simulink model "Boat_model_paper"  (Simulink 6.6)
settings: Solver=ode3  StartTime=0.0  StopTime=500  FixedStep=.01  RelTol=1e-3
values from neighbouring files (symbols this model uses):
  C_d_sea_surge = -340    [boat_constants.m]
  C_F = 1.15    [boat_constants.m]
  C_T = 6.4/(pi*rho_w*rudder_span*d_prop)    (= 0.00946194530212)    [boat_constants.m]
  d_prop = .4572    (= 0.4572)    [boat_constants.m]
  delta_stall = .279    (= 0.279)    [boat_constants.m]
  e_0 = 0    [boat_constants.m]
  I_xx = mass/12*(3^2+4^2)    (= 1145.83333333)    [boat_constants.m]
  I_zz = mass/12*(13^2+3^2)    (= 8158.33333333)    [boat_constants.m]
  K_t = 0.5    [boat_constants.m]
  mass = 550    [boat_constants.m]
  n_0 = 0    [boat_constants.m]
  proportional_band = .5    (= 0.5)    [boat_constants.m]
  psi_0 = 0    [boat_constants.m]
  rho_w = 1.03e3    (= 1030)    [boat_constants.m]
  rudder_angle_dot_max = 10    [boat_constants.m]
  rudder_angle_max = 1    [boat_constants.m]
  rudder_area = .0945    (= 0.0945)    [boat_constants.m]
  Wf = 1 - Wt    (= 0.9)    [boat_constants.m]
  x_cg = .0508    (= 0.0508)    [boat_constants.m]
  x_cp = 3.4224    [boat_constants.m]
  z_cg = .0508    (= 0.0508)    [boat_constants.m]
  z_cp = .2032    (= 0.2032)    [boat_constants.m]
undefined symbols (not defined in the file or in its folder): render_boat
libraries: simulink x4, vrlib x1
settings Model: Creator=Administrator  LastModifiedBy=Administrator  SimulationMode=accelerator
settings DebuggingCC: AlgebraicLoopMsg=error

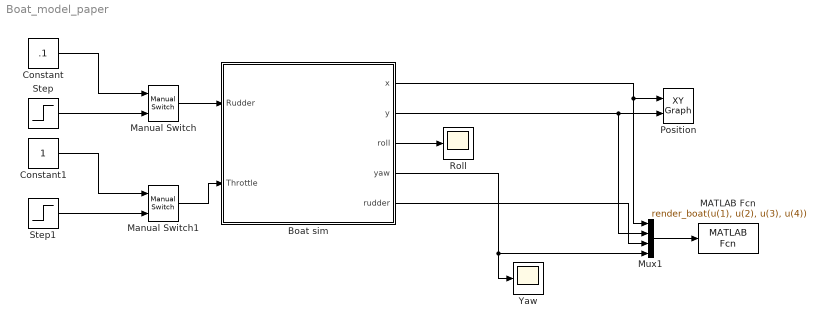
== system Boat_model_paper ==
  Boat sim : Subsystem
  Constant : Constant  Value=.1
  Constant1 : Constant
  MATLAB Fcn : MATLABFcn  MATLABFcn=render_boat(u(1), u(2), u(3), u(4))  OutputDimensions=0
  Manual Switch : simulink/Signal Routing/Manual Switch  SystemSampleTime=-1  sw=1  action=0  varsize=off
  Manual Switch1 : simulink/Signal Routing/Manual Switch  SystemSampleTime=-1  sw=1  action=0  varsize=off
  Mux1 : Mux
  Position : simulink/Sinks/XY Graph  SystemSampleTime=-1  xmin=-1000  xmax=1000  ymin=-1000  ymax=1000  st=-1
  Roll : Scope
  Step : Step  Time=5  SampleTime=0
  Step1 : Step  Time=5  SampleTime=0
  Yaw : Scope
      settings: SaveName=ScopeData4
  wires:
  Mux1/1 -> MATLAB Fcn/1
  Boat sim/1(x) -> Mux1/1, Position/1
  Boat sim/2(y) -> Position/2, Mux1/2
  Boat sim/4(yaw) -> Mux1/4, Yaw/1
  Boat sim/3(roll) -> Roll/1
  Boat sim/5(rudder) -> Mux1/3
  Step/1 -> Manual Switch/2
  Manual Switch/1 -> Boat sim/1(Rudder)
  Constant/1 -> Manual Switch/1
  Step1/1 -> Manual Switch1/2
  Manual Switch1/1 -> Boat sim/2(Throttle)
  Constant1/1 -> Manual Switch1/1

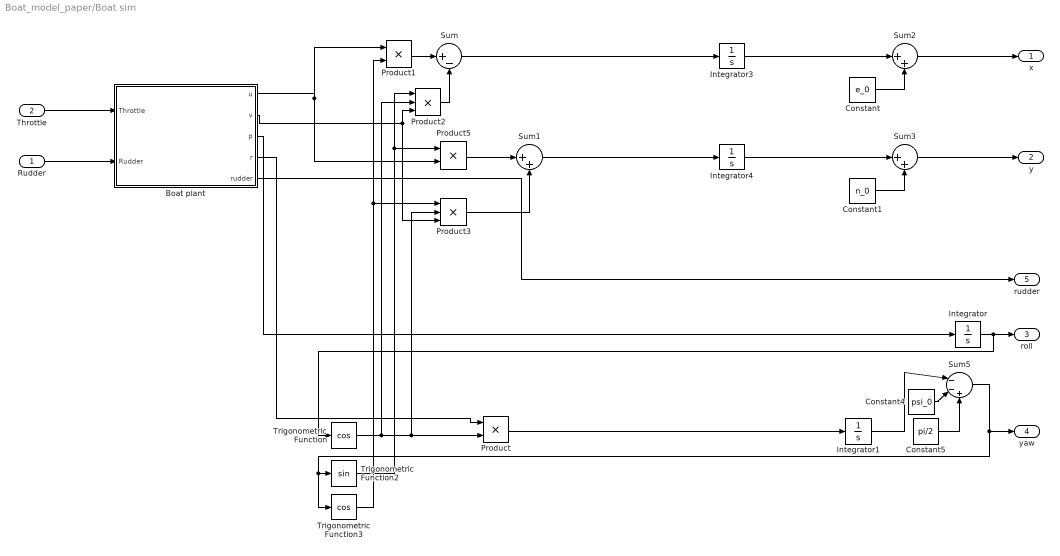
== system Boat_model_paper/Boat sim ==
  Rudder : Inport
  Throttle : Inport  Port=2
  Boat plant : Subsystem
  Constant : Constant  Value=e_0
  Constant1 : Constant  Value=n_0
  Constant4 : Constant  Value=psi_0
  Constant5 : Constant  Value=pi/2
  Integrator{,1,3..4} (4 alike) : Integrator
  Product : Product  RndMeth=Zero
  Product1 : Product  RndMeth=Zero
  Product2 : Product  Inputs=3  RndMeth=Zero
  Product3 : Product  Inputs=3  RndMeth=Zero
  Product5 : Product  RndMeth=Zero
  Sum : Sum  Inputs=|+-
  Sum1 : Sum  Inputs=|++
  Sum2 : Sum  Inputs=|++
  Sum3 : Sum  Inputs=|++
  Sum5 : Sum  Inputs=|--+
  Trigonometric Function : Trigonometry  Operator=cos
  Trigonometric Function2 : Trigonometry
  Trigonometric Function3 : Trigonometry  Operator=cos
  x : Outport
  y : Outport  Port=2
  roll : Outport  Port=3
  yaw : Outport  Port=4
  rudder : Outport  Port=5
  wires:
  Throttle/1 -> Boat plant/1(Throttle)
  Rudder/1 -> Boat plant/2(Rudder)
  Boat plant/3(p) -> Integrator/1
  Trigonometric Function/1 -> Product/2, Product3/2, Product2/2
  Boat plant/4(r) -> Product/1
  Product/1 -> Integrator1/1
  Product2/1 -> Sum/2
  Product1/1 -> Sum/1
  Boat plant/1(u) -> Product1/1, Product5/2
  Trigonometric Function3/1 -> Product1/2, Product3/1
  Trigonometric Function2/1 -> Product2/1, Product5/1
  Boat plant/2(v) -> Product2/3, Product3/3
  Product5/1 -> Sum1/1
  Product3/1 -> Sum1/2
  Sum/1 -> Integrator3/1
  Integrator/1 -> roll/1, Trigonometric Function/1
  Constant4/1 -> Sum5/2
  Constant5/1 -> Sum5/3
  Integrator1/1 -> Sum5/1
  Sum5/1 -> yaw/1, Trigonometric Function2/1, Trigonometric Function3/1
  Boat plant/5(rudder) -> rudder/1
  Constant/1 -> Sum2/2
  Integrator3/1 -> Sum2/1
  Sum2/1 -> x/1
  Integrator4/1 -> Sum3/1
  Constant1/1 -> Sum3/2
  Sum3/1 -> y/1
  Sum1/1 -> Integrator4/1

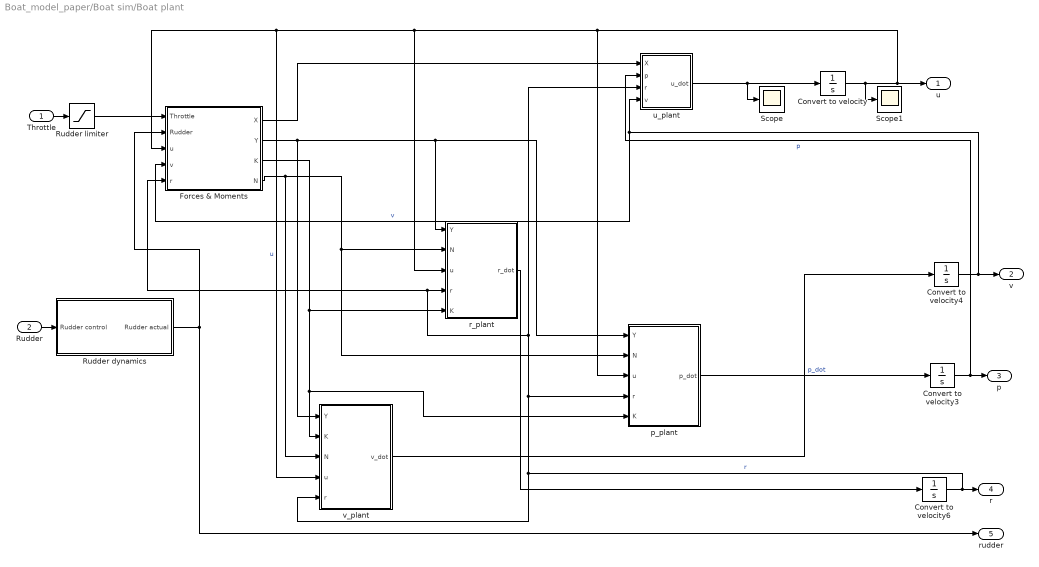
== system Boat_model_paper/Boat sim/Boat plant ==
  Throttle : Inport
  Rudder : Inport  Port=2
  Convert to velocity{,3..4,6} (4 alike) : Integrator
  Forces & Moments : Subsystem
  Rudder dynamics : Subsystem
  Rudder limiter : Saturate  UpperLimit=1  LowerLimit=0
  Scope : Scope
      settings: SaveName=ScopeData2
  Scope1 : Scope
      settings: SaveName=ScopeData3
  p_plant : Subsystem
  r_plant : Subsystem
  u_plant : Subsystem
  v_plant : Subsystem
  u : Outport
  v : Outport  Port=2
  p : Outport  Port=3
  r : Outport  Port=4
  rudder : Outport  Port=5
  wires:
  Convert to velocity/1 -> u/1, r_plant/3(u), Forces & Moments/3(u), v_plant/4(u), p_plant/3(u), Scope1/1  "u"
  Forces & Moments/1(X) -> u_plant/1(X)
  Rudder/1 -> Rudder dynamics/1(Rudder control)
  Throttle/1 -> Rudder limiter/1
  Convert to velocity4/1 -> v/1, u_plant/4(v), Forces & Moments/4(v)  "v"
  p_plant/1(p_dot) -> Convert to velocity3/1  "p_dot"
  Convert to velocity3/1 -> p/1, u_plant/2(p)  "p"
  Convert to velocity6/1 -> r/1, v_plant/5(r), u_plant/3(r), r_plant/4(r), Forces & Moments/5(r), p_plant/4(r)  "r"
  u_plant/1(u_dot) -> Convert to velocity/1, Scope/1
  Forces & Moments/4(N) -> v_plant/3(N), r_plant/2(N), p_plant/2(N)
  Forces & Moments/3(K) -> v_plant/2(K), p_plant/5(K), r_plant/5(K)
  Forces & Moments/2(Y) -> v_plant/1(Y), r_plant/1(Y), p_plant/1(Y)
  v_plant/1(v_dot) -> Convert to velocity4/1
  r_plant/1(r_dot) -> Convert to velocity6/1
  Rudder limiter/1 -> Forces & Moments/1(Throttle)
  Rudder dynamics/1(Rudder actual) -> Forces & Moments/2(Rudder), rudder/1

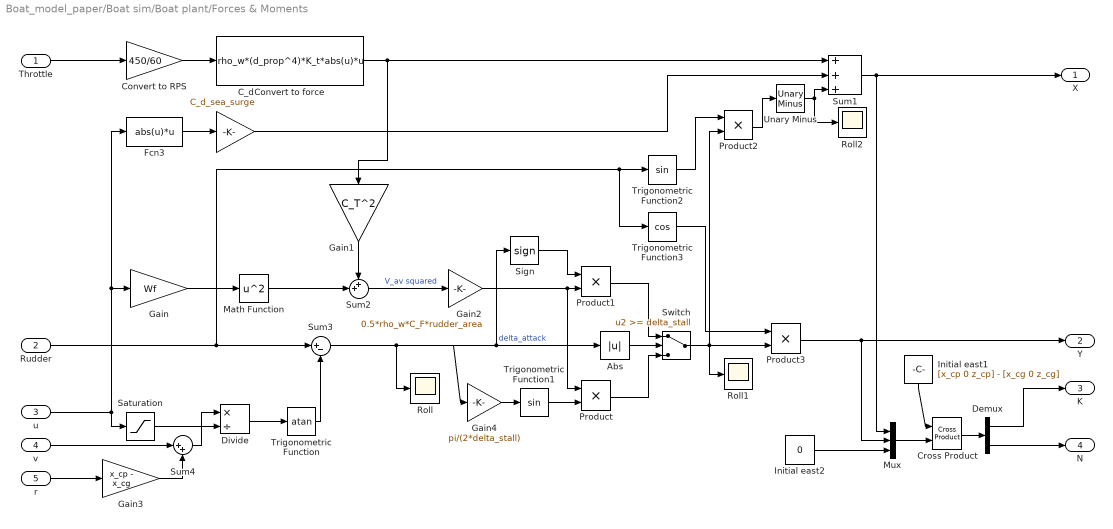
== system Boat_model_paper/Boat sim/Boat plant/Forces & Moments ==
  Throttle : Inport
  Rudder : Inport  Port=2
  u : Inport  Port=3
  v : Inport  Port=4
  r : Inport  Port=5
  Abs : Abs
  C_d : Gain  Gain=C_d_sea_surge
  Convert to RPS : Gain  Gain=450/60
  Convert to force : Fcn  Expr=rho_w*(d_prop^4)*K_t*abs(u)*u
  Cross Product : vrlib/Utilities/Cross Product  SystemSampleTime=-1
  Demux : Demux  Outputs=3
  Divide : Product  Inputs=*/  OutScaling=2^-10
  Fcn3 : Fcn  Expr=abs(u)*u
  Gain : Gain  Gain=Wf
  Gain1 : Gain  Orientation=down  Gain=C_T^2
  Gain2 : Gain  Gain=0.5*rho_w*C_F*rudder_area
  Gain3 : Gain  Gain=x_cp - x_cg
  Gain4 : Gain  Gain=pi/(2*delta_stall)
  Initial east1 : Constant  Orientation=down  Value=[x_cp 0 z_cp] - [x_cg 0 z_cg]
  Initial east2 : Constant  Value=0
  Math Function : Math  Operator=square  SaturateOnIntegerOverflow=on
  Mux : Mux  Inputs=3
  Product{,1..3} (4 alike) : Product  RndMeth=Zero
  Roll : Scope
  Roll1 : Scope
      settings: SaveName=ScopeData5
  Roll2 : Scope
      settings: SaveName=ScopeData6
  Saturation : Saturate  UpperLimit=inf  LowerLimit=0.00001
  Sign : Signum
  Sum1 : Sum  Inputs=+++
  Sum2 : Sum  Inputs=++|
  Sum3 : Sum  Inputs=|+-
  Sum4 : Sum  Inputs=|++
  Switch : Switch  Threshold=delta_stall
  Trigonometric Function : Trigonometry  Operator=atan
  Trigonometric Function1 : Trigonometry
  Trigonometric Function2 : Trigonometry
  Trigonometric Function3 : Trigonometry  Operator=cos
  Unary Minus : simulink/Math Operations/Unary Minus  DoSatur=off
  X : Outport
  Y : Outport  Port=2
  K : Outport  Port=3
  N : Outport  Port=4
  wires:
  Convert to RPS/1 -> Convert to force/1
  Fcn3/1 -> C_d/1
  C_d/1 -> Sum1/2
  Convert to force/1 -> Sum1/1, Gain1/1
  u/1 -> Fcn3/1, Gain/1, Saturation/1
  Throttle/1 -> Convert to RPS/1
  Sum1/1 -> X/1, Mux/1
  Gain/1 -> Math Function/1
  Gain1/1 -> Sum2/1
  Math Function/1 -> Sum2/2
  Sum2/1 -> Gain2/1  "V_av squared"
  Rudder/1 -> Sum3/1, Trigonometric Function2/1, Trigonometric Function3/1
  r/1 -> Gain3/1
  Gain3/1 -> Sum4/2
  v/1 -> Sum4/1
  Divide/1 -> Trigonometric Function/1
  Sum4/1 -> Divide/1
  Trigonometric Function/1 -> Sum3/2
  Sum3/1 -> Abs/1, Sign/1, Gain4/1, Roll/1  "delta_attack"
  Abs/1 -> Switch/2
  Product/1 -> Switch/3
  Trigonometric Function1/1 -> Product/2
  Gain2/1 -> Product/1, Product1/2
  Product1/1 -> Switch/1
  Sign/1 -> Product1/1
  Gain4/1 -> Trigonometric Function1/1
  Unary Minus/1 -> Sum1/3, Roll2/1
  Product2/1 -> Unary Minus/1
  Trigonometric Function2/1 -> Product2/1
  Trigonometric Function3/1 -> Product3/1
  Product3/1 -> Y/1, Mux/2
  Cross Product/1 -> Demux/1
  Demux/1 -> K/1
  Demux/3 -> N/1
  Switch/1 -> Product2/2, Product3/2, Roll1/1
  Saturation/1 -> Divide/2
  Initial east2/1 -> Mux/3
  Mux/1 -> Cross Product/2
  Initial east1/1 -> Cross Product/1

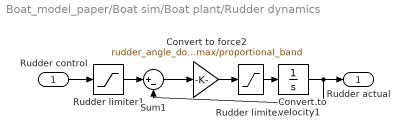
== system Boat_model_paper/Boat sim/Boat plant/Rudder dynamics ==
  Rudder control : Inport
  Convert to force2 : Gain  Gain=rudder_angle_dot_max/proportional_band
  Convert to velocity1 : Integrator  LimitOutput=on  UpperSaturationLimit=rudder_angle_max  LowerSaturationLimit=-rudder_angle_max
  Rudder limiter1 : Saturate  UpperLimit=rudder_angle_max  LowerLimit=-rudder_angle_max
  Rudder limiter2 : Saturate  UpperLimit=rudder_angle_dot_max  LowerLimit=-rudder_angle_dot_max
  Sum1 : Sum  Inputs=|+-
  Rudder actual : Outport
  wires:
  Convert to velocity1/1 -> Rudder actual/1, Sum1/2
  Sum1/1 -> Convert to force2/1
  Rudder limiter1/1 -> Sum1/1
  Rudder limiter2/1 -> Convert to velocity1/1
  Convert to force2/1 -> Rudder limiter2/1
  Rudder control/1 -> Rudder limiter1/1

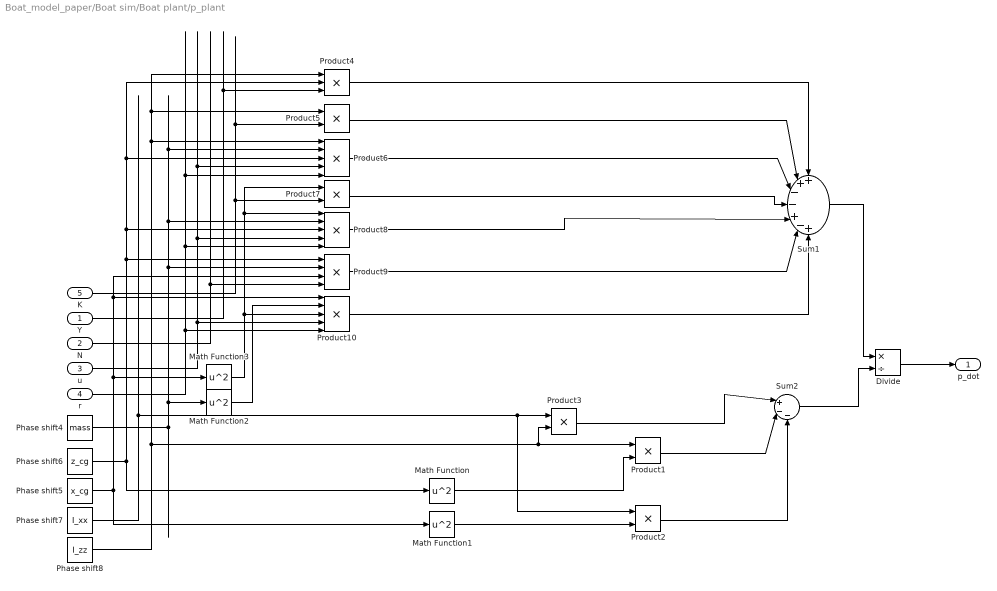
== system Boat_model_paper/Boat sim/Boat plant/p_plant ==
  Y : Inport
  N : Inport  Port=2
  u : Inport  Port=3
  r : Inport  Port=4
  K : Inport  Port=5
  Divide : Product  Inputs=*/  OutScaling=2^-10
  Math Function{,1..3} (4 alike) : Math  Operator=square  SaturateOnIntegerOverflow=on
  Phase shift4 : Constant  Value=mass
  Phase shift5 : Constant  Value=x_cg
  Phase shift6 : Constant  Value=z_cg
  Phase shift7 : Constant  Value=I_xx
  Phase shift8 : Constant  Value=I_zz
  Product{1..3,5,7} (5 alike) : Product  RndMeth=Zero
  Product10 : Product  Inputs=5  RndMeth=Zero
  Product4 : Product  Inputs=3  RndMeth=Zero
  Product6 : Product  Inputs=5  RndMeth=Zero
  Product8 : Product  Inputs=5  RndMeth=Zero
  Product9 : Product  Inputs=4  RndMeth=Zero
  Sum1 : Sum  Inputs=++--+-+
  Sum2 : Sum  Inputs=|+--
  p_dot : Outport
  wires:
  Sum1/1 -> Divide/1
  Divide/1 -> p_dot/1
  r/1 -> Product6/5, Product8/5, Product10/5
  u/1 -> Product6/4, Product8/4, Product10/4
  N/1 -> Product9/4
  Y/1 -> Product4/3
  Sum2/1 -> Divide/2
  Phase shift7/1 -> Product3/1, Product2/1
  Phase shift8/1 -> Product3/2, Product1/1, Product4/1, Product5/1, Product6/1
  Product3/1 -> Sum2/1
  Phase shift6/1 -> Math Function/1, Product4/2, Product6/3, Product8/3, Product9/1
  Math Function/1 -> Product1/2
  Product1/1 -> Sum2/2
  Math Function1/1 -> Product2/2
  Product2/1 -> Sum2/3
  Phase shift4/1 -> Product6/2, Product8/2, Product9/2, Math Function2/1
  K/1 -> Product5/2, Product7/2
  Phase shift5/1 -> Math Function1/1, Math Function3/1, Product9/3, Product10/1
  Product4/1 -> Sum1/1
  Product5/1 -> Sum1/2
  Product6/1 -> Sum1/3
  Product7/1 -> Sum1/4
  Math Function3/1 -> Product7/1, Product8/1, Product10/3
  Product8/1 -> Sum1/5
  Product9/1 -> Sum1/6
  Product10/1 -> Sum1/7
  Math Function2/1 -> Product10/2

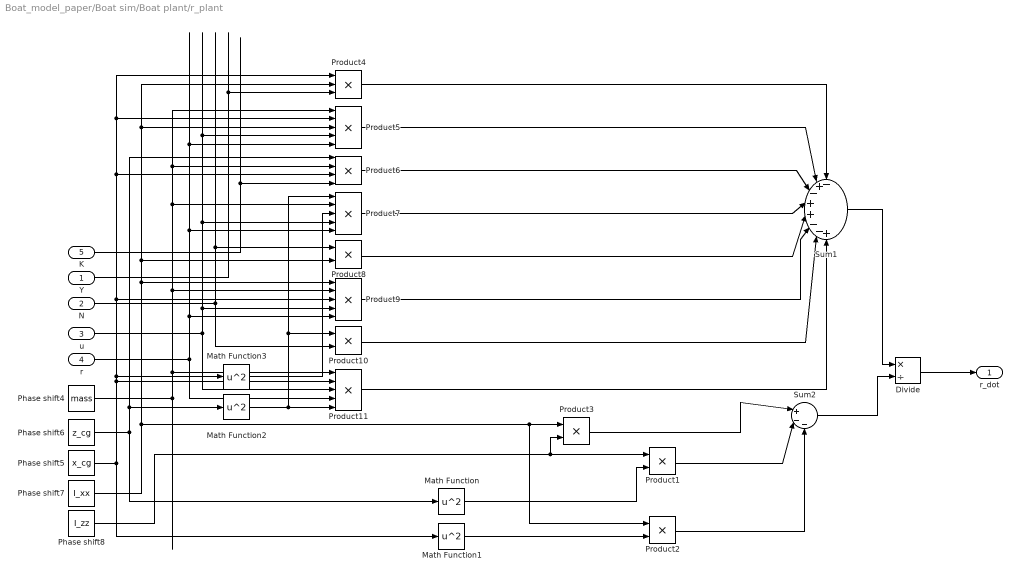
== system Boat_model_paper/Boat sim/Boat plant/r_plant ==
  Y : Inport
  N : Inport  Port=2
  u : Inport  Port=3
  r : Inport  Port=4
  K : Inport  Port=5
  Divide : Product  Inputs=*/  OutScaling=2^-10
  Math Function{,1..3} (4 alike) : Math  Operator=square  SaturateOnIntegerOverflow=on
  Phase shift4 : Constant  Value=mass
  Phase shift5 : Constant  Value=x_cg
  Phase shift6 : Constant  Value=z_cg
  Phase shift7 : Constant  Value=I_xx
  Phase shift8 : Constant  Value=I_zz
  Product{1..3,8,10} (5 alike) : Product  RndMeth=Zero
  Product{5,7,9,11} (4 alike) : Product  Inputs=5  RndMeth=Zero
  Product4 : Product  Inputs=3  RndMeth=Zero
  Product6 : Product  Inputs=4  RndMeth=Zero
  Sum1 : Sum  Inputs=-+-++--+
  Sum2 : Sum  Inputs=|+--
  r_dot : Outport
  wires:
  Sum1/1 -> Divide/1
  Divide/1 -> r_dot/1
  r/1 -> Product5/5, Product7/5, Product9/5, Product11/4
  u/1 -> Product5/4, Product7/4, Product9/4, Product11/3
  N/1 -> Product8/1, Product10/2
  Y/1 -> Product4/3
  Sum2/1 -> Divide/2
  Phase shift7/1 -> Product3/1, Product2/1, Product4/2, Product5/3, Product8/2, Product9/1
  Phase shift8/1 -> Product3/2, Product1/1
  Product3/1 -> Sum2/1
  Phase shift6/1 -> Math Function/1, Product6/1, Math Function2/1
  Math Function/1 -> Product1/2
  Product1/1 -> Sum2/2
  Math Function1/1 -> Product2/2
  Phase shift5/1 -> Math Function1/1, Product4/1, Product5/2, Product6/3, Product9/3, Math Function3/1, Product11/2
  Product2/1 -> Sum2/3
  Phase shift4/1 -> Product5/1, Product6/2, Product7/2, Product9/2, Product11/1
  Product4/1 -> Sum1/1
  Product5/1 -> Sum1/2
  Product6/1 -> Sum1/3
  K/1 -> Product6/4
  Product7/1 -> Sum1/4
  Math Function2/1 -> Product7/1, Product10/1, Product11/5
  Product8/1 -> Sum1/5
  Product9/1 -> Sum1/6
  Product10/1 -> Sum1/7
  Product11/1 -> Sum1/8
  Math Function3/1 -> Product7/3

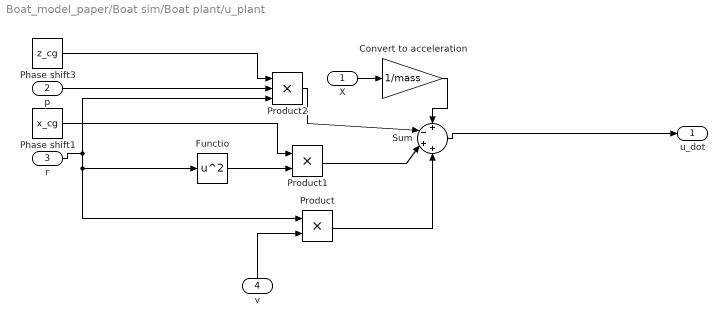
== system Boat_model_paper/Boat sim/Boat plant/u_plant ==
  X : Inport
  p : Inport  Port=2
  r : Inport  Port=3
  v : Inport  Orientation=up  Port=4
  Convert to acceleration : Gain  Gain=1/mass
  Functio : Math  Operator=square  SaturateOnIntegerOverflow=on
  Phase shift1 : Constant  Value=x_cg
  Phase shift3 : Constant  Value=z_cg
  Product : Product  RndMeth=Zero
  Product1 : Product  RndMeth=Zero
  Product2 : Product  Inputs=3  RndMeth=Zero
  Sum : Sum  Inputs=+-++
  u_dot : Outport
  wires:
  Product/1 -> Sum/4
  Functio/1 -> Product1/2
  Product1/1 -> Sum/3
  Product2/1 -> Sum/2
  Phase shift3/1 -> Product2/1
  p/1 -> Product2/2
  Phase shift1/1 -> Product1/1
  r/1 -> Product/1, Product2/3, Functio/1
  v/1 -> Product/2
  Sum/1 -> u_dot/1
  Convert to acceleration/1 -> Sum/1
  X/1 -> Convert to acceleration/1

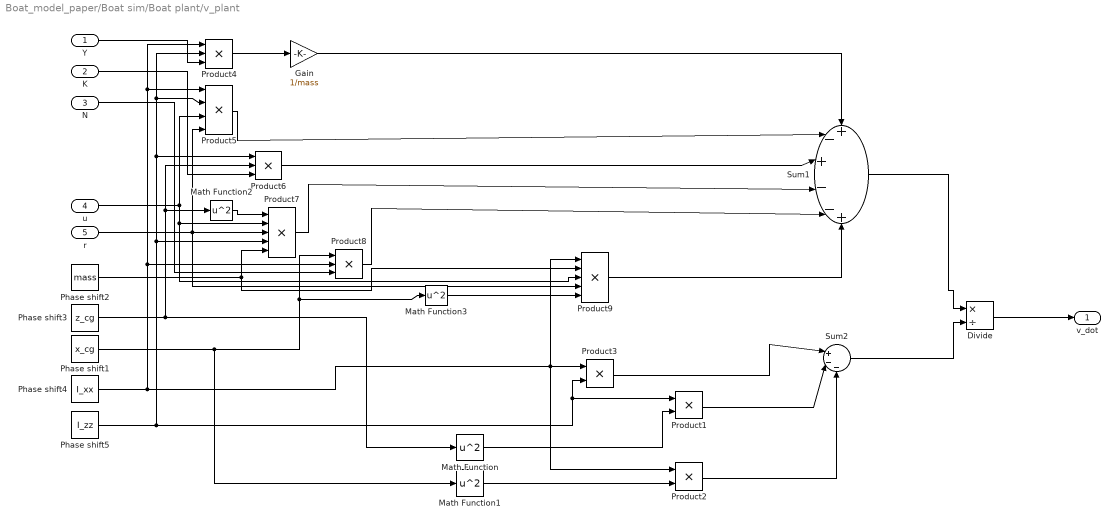
== system Boat_model_paper/Boat sim/Boat plant/v_plant ==
  Y : Inport
  K : Inport  Port=2
  N : Inport  Port=3
  u : Inport  Port=4
  r : Inport  Port=5
  Divide : Product  Inputs=*/  OutScaling=2^-10
  Gain : Gain  Gain=1/mass
  Math Function{,1..3} (4 alike) : Math  Operator=square  SaturateOnIntegerOverflow=on
  Phase shift1 : Constant  Value=x_cg
  Phase shift2 : Constant  Value=mass
  Phase shift3 : Constant  Value=z_cg
  Phase shift4 : Constant  Value=I_xx
  Phase shift5 : Constant  Value=I_zz
  Product1 : Product  RndMeth=Zero
  Product2 : Product  RndMeth=Zero
  Product3 : Product  RndMeth=Zero
  Product4 : Product  Inputs=3  RndMeth=Zero
  Product5 : Product  Inputs=4  RndMeth=Zero
  Product6 : Product  Inputs=3  RndMeth=Zero
  Product7 : Product  Inputs=5  RndMeth=Zero
  Product8 : Product  Inputs=3  RndMeth=Zero
  Product9 : Product  Inputs=5  RndMeth=Zero
  Sum1 : Sum  Inputs=+-+--+
  Sum2 : Sum  Inputs=|+--
  v_dot : Outport
  wires:
  Divide/1 -> v_dot/1
  Sum2/1 -> Divide/2
  Phase shift4/1 -> Product3/1, Product2/1, Product9/1, Product4/1, Product5/1, Product8/2
  Phase shift5/1 -> Product3/2, Product1/1, Product4/2, Product5/2, Product6/1, Product7/4
  Product3/1 -> Sum2/1
  Phase shift3/1 -> Math Function/1, Product6/2, Math Function2/1
  Math Function/1 -> Product1/2
  Product1/1 -> Sum2/2
  Math Function1/1 -> Product2/2
  Phase shift1/1 -> Math Function1/1, Product8/1, Math Function3/1
  Product2/1 -> Sum2/3
  Y/1 -> Product4/3
  Product4/1 -> Gain/1
  Gain/1 -> Sum1/1
  u/1 -> Product5/3, Product7/2, Product9/3
  r/1 -> Product5/4, Product7/3, Product9/4
  Product5/1 -> Sum1/2
  Product6/1 -> Sum1/3
  K/1 -> Product6/3
  Phase shift2/1 -> Product7/5, Product9/2
  Math Function2/1 -> Product7/1
  Product7/1 -> Sum1/4
  Product8/1 -> Sum1/5
  N/1 -> Product8/3
  Product9/1 -> Sum1/6
  Math Function3/1 -> Product9/5
  Sum1/1 -> Divide/1
